simulink model "BD_SER2"  (Simulink 4.1.1)
settings: Solver=ode1  SolverMode=SingleTasking  StartTime=0.0  StopTime=max(cyc_mph(:,1))  FixedStep=1  MaxStep=1  RelTol=1e-3  AbsTol=1e-3
undefined symbols (not defined in the file): air_cp, amb_tmp, cyc_avg_time, cyc_cargo_mass, cyc_elevation_init, cyc_filter_bool, cyc_grade, cyc_mph, enable_stop, ess_cap_scale, ess_coulombic_eff, ess_init_soc, ess_max_ah_cap, ess_max_volts, ess_min_volts, ess_mod_airflow, ess_mod_cp, ess_mod_init_tmp, ess_module_mass, ess_module_num, ess_on, ess_res_scale_coef, ess_res_scale_fun, ess_set_tmp, ess_th_calc, ess_th_res_off, ess_th_res_on, ess_tmp, ess_voc, ex_calc, fc_ct_trq, fc_emis, fc_inertia, fc_map_spd, fc_max_trq, fc_spd_scale, fc_trq_scale, fd_inertia, fd_loss, fd_ratio, gb_dnshift_load, gb_dnshift_spd, gb_gears_num, gb_inertia, gb_num_init, gb_ratio, gb_shift_delay, gb_spd_scale, gb_trq_scale, gb_upshift_load, gb_upshift_spd, gc_inertia, gc_map_spd, gc_map_trq, gc_max_crrnt, gc_max_trq, gc_outpwr_map, gc_overtrq_factor, gc_spd_scale, gc_trq_scale ... (+37)
libraries: lib_wheel2 x12, lib_accessory2 x4, lib_controls2 x3, lib_etc x2, lib_help x2, lib_fuel_converter x2, lib_drive_cycle2 x1, lib_interactive x1, lib_drive_cycle x1, lib_exhaust x1, lib_fuel_converter3 x1
(part 11 of 15)

== system BD_SER2/final drive <fd>/model&interface/model/enhancedToWorkspace4 ==
  In1 : Inport  Port=1  LatchInput=off
  To Workspace : ToWorkspace  VariableName=fd_spd_in_r  SampleTime=-1  SaveFormat=Array
  wires:
  In1/1 -> To Workspace/1

== system BD_SER2/final drive <fd>/model&interface/model/enhancedToWorkspace5 ==
  In1 : Inport  Port=1  LatchInput=off
  To Workspace : ToWorkspace  VariableName=fd_trq_in_r  SampleTime=-1  SaveFormat=Array
  wires:
  In1/1 -> To Workspace/1

== system BD_SER2/final drive <fd>/model&interface/model/enhancedToWorkspace6 ==
  In1 : Inport  Port=1  LatchInput=off
  To Workspace : ToWorkspace  VariableName=fd_trq_out_r  SampleTime=-1  SaveFormat=Array
  wires:
  In1/1 -> To Workspace/1

== system BD_SER2/final drive <fd>/model&interface/model/enhancedToWorkspace7 ==
  In1 : Inport  Port=1  LatchInput=off
  To Workspace : ToWorkspace  VariableName=fd_spd_out_r  SampleTime=-1  SaveFormat=Array
  wires:
  In1/1 -> To Workspace/1

== system BD_SER2/final drive <fd>/model&interface/model/help ==

== system BD_SER2/final drive <fd>/model&interface/model/loss (Nm) ==
  note: The loss torque is zero when the gears are not turning,
      | and is applied at the input side of the gear reduction.
  fd output speed (rad/s) : Inport  Port=1  LatchInput=off
  Constant : Constant  Orientation=up  Value=0
  Switch : Switch  Threshold=eps
  final drive loss torque (Nm) : Constant  Value=fd_loss
  drag torque (Nm) : Outport  Port=1  InitialOutput=0
  wires:
  Constant/1 -> Switch/3
  fd output speed (rad/s)/1 -> Switch/2
  Switch/1 -> drag torque (Nm)/1
  final drive loss torque (Nm)/1 -> Switch/1

== system BD_SER2/fuel converter  <fc> for series/Model & Interface/model/Block NOTES ==
  note: This block models the internal combustion engine, and includes inertia effects,
      | performance limits, accessory loads, and temperature transient effects on fuel
      | use, engine-out emissions, and catalyst efficiency.  There are 'leads' to the
      | engine controller here, which controller determines whether the engine is on.

== system BD_SER2/fuel converter  <fc> for series/Model & Interface/model/enhancedToWorkspace ==
  In1 : Inport  Port=1  LatchInput=off
  To Workspace : ToWorkspace  VariableName=fc_spd_out_r  SampleTime=-1  SaveFormat=Array
  wires:
  In1/1 -> To Workspace/1

== system BD_SER2/fuel converter  <fc> for series/Model & Interface/model/enhancedToWorkspace1 ==
  In1 : Inport  Port=1  LatchInput=off
  To Workspace : ToWorkspace  VariableName=fc_trq_out_r  SampleTime=-1  SaveFormat=Array
  wires:
  In1/1 -> To Workspace/1

== system BD_SER2/fuel converter  <fc> for series/Model & Interface/model/enhancedToWorkspace2 ==
  In1 : Inport  Port=1  LatchInput=off
  To Workspace : ToWorkspace  VariableName=fc_spd_est  SampleTime=-1  SaveFormat=Array
  wires:
  In1/1 -> To Workspace/1

== system BD_SER2/fuel converter  <fc> for series/Model & Interface/model/enhancedToWorkspace3 ==
  In1 : Inport  Port=1  LatchInput=off
  To Workspace : ToWorkspace  VariableName=fc_brake_trq  SampleTime=-1  SaveFormat=Array
  wires:
  In1/1 -> To Workspace/1

== system BD_SER2/fuel converter  <fc> for series/Model & Interface/model/enhancedToWorkspace4 ==
  In1 : Inport  Port=1  LatchInput=off
  To Workspace : ToWorkspace  VariableName=fc_trq_out_a  SampleTime=-1  SaveFormat=Array
  wires:
  In1/1 -> To Workspace/1

== system BD_SER2/fuel converter  <fc> for series/Model & Interface/model/enhancedToWorkspace5 ==
  In1 : Inport  Port=1  LatchInput=off
  To Workspace : ToWorkspace  VariableName=fc_spd_out_a  SampleTime=-1  SaveFormat=Array
  wires:
  In1/1 -> To Workspace/1

== system BD_SER2/fuel converter  <fc> for series/Model & Interface/model/fuel use and EO emis Configurable Subsystem ==
  T (Nm) : Inport  Port=1  LatchInput=off
  w (rad/s) : Inport  Port=2  LatchInput=off
  fuel use and EO emis : lib_fuel_converter3/configurable subsystems/fuel use and EO emis
      settings: RTWFcnNameOpts=Auto  RTWFileNameOpts=Auto
  cumulative fuel  use (gal) : Outport  Port=1
  "FC ON?, EOem, MFex, Tex, O2ex" : Outport  Port=2
  Vv,Tfc : Outport  Port=3
  wires:
  T (Nm)/1 -> fuel use and EO emis/1
  w (rad/s)/1 -> fuel use and EO emis/2
  fuel use and EO emis/1 -> cumulative fuel  use (gal)/1
  fuel use and EO emis/2 -> "FC ON?, EOem, MFex, Tex, O2ex"/1
  fuel use and EO emis/3 -> Vv,Tfc/1

== system BD_SER2/fuel converter  <fc> for series/Model & Interface/model/help ==

== system BD_SER2/fuel converter  <fc> for series/Model & Interface/model/providing trq (+ive or -ive) ==
  req'd trq (Nm) : Inport  Port=1  LatchInput=off
  req'd spd (rad/s) : Inport  Port=2  LatchInput=off
  prev engine spd (rad/s) : Inport  Port=3  LatchInput=off
  Mux3 : Mux  Inputs=3
      settings: DisplayOption=none
  Sum1 : Sum  Inputs=+-  SaturateOnIntegerOverflow=on
  Sum2 : Sum  Inputs=++  SaturateOnIntegerOverflow=on
  effect of inertia (Nm) : Subsystem
      settings: RTWFcnNameOpts=Auto  RTWFileNameOpts=Auto
  enforce engine limits : Subsystem
      settings: RTWFcnNameOpts=Auto  RTWFileNameOpts=Auto
  map trq (Nm) spd (rad/s) trq to drivetrain (Nm) : Outport  Port=1  InitialOutput=0
  wires:
  Sum2/1 -> enforce engine limits/1(req'd engine trq (Nm))
  effect of inertia (Nm)/1((Nm)) -> Sum2/2, Sum1/2
  req'd trq (Nm)/1 -> Sum2/1
  enforce engine limits/2(limited engine spd (rad/s)) -> Mux3/2, effect of inertia (Nm)/1(req'd spd (rad/s))
  enforce engine limits/1(limited engine brake trq (Nm)) -> Sum1/1, Mux3/1
  prev engine spd (rad/s)/1 -> effect of inertia (Nm)/2(prev spd)
  Mux3/1 -> map trq (Nm) spd (rad/s) trq to drivetrain (Nm)/1
  Sum1/1 -> Mux3/3
  req'd spd (rad/s)/1 -> enforce engine limits/2(req'd engine spd (rad/s))

== system BD_SER2/fuel converter  <fc> for series/Model & Interface/model/spinning up or spinning down ==
  spd command (rad/s) : Inport  Port=1  LatchInput=off
  engine disconnected from drivetrain : Inport  Port=2  LatchInput=off
  previous engine spd (rad/s) : Inport  Port=3  LatchInput=off
  Constant : Constant  Value=0
  Constant1 : Constant  Value=vc_idle_spd
  MinMax : MinMax  Function=min  Inputs=2
  MinMax1 : MinMax  Function=max  Inputs=2
  Mux3 : Mux  Inputs=3
      settings: DisplayOption=none
  Product : Product  Inputs=2  Multiplication=Element-wise(.*)  SaturateOnIntegerOverflow=on
  Product2 : Product  Inputs=2  Multiplication=Element-wise(.*)  SaturateOnIntegerOverflow=on
  Relational Operator : RelationalOperator  Operator=<=
  Sum : Sum  Inputs=|++  SaturateOnIntegerOverflow=on
  Sum1 : Sum  Inputs=|+-  SaturateOnIntegerOverflow=on
  Sum2 : Sum  Inputs=++  SaturateOnIntegerOverflow=on
  Switch: map torque : Switch  Threshold=eps
  T_closed throttle : Subsystem
      settings: RTWFcnNameOpts=Auto  RTWFileNameOpts=Auto
  T_max : Subsystem
      settings: RTWFcnNameOpts=Auto  RTWFileNameOpts=Auto
  alpha : Gain  Gain=1/(fc_inertia+eps)  Multiplication=Element-wise(K.*u)  SaturateOnIntegerOverflow=on
  dt : Subsystem
      settings: RTWFcnNameOpts=Auto  RTWFileNameOpts=Auto
  effect of inertia (Nm) : Subsystem
      settings: RTWFcnNameOpts=Auto  RTWFileNameOpts=Auto
  just started spin-down/spin-up : Subsystem
      settings: RTWFcnNameOpts=Auto  RTWFileNameOpts=Auto
  no-lag Reset Integrator : Subsystem  mask(No-lag Reset Integrator){@1=vc_idle_spd}
      mask prompts: @1 "Initial Value"
      mask help: No-lag Reset Integrator
      mask init:
      | initval=@1;
      settings: RTWFcnNameOpts=Auto  RTWFileNameOpts=Auto
      mask Help: Integrates first input using Euler technique.\nAt the time step that input 2 <> zero,\noutput is reset to input 3.
      mask Display: disp('1/s\nw/ reset\nno lag')
  map trq (Nm) spd (rad/s) trq to drivetrain (Nm) : Outport  Port=1  InitialOutput=0
  wires:
  T_max/1(T_max) -> MinMax/1
  MinMax/1 -> Switch: map torque/1
  T_closed throttle/1(T_closed throttle) -> Switch: map torque/3
  Switch: map torque/1 -> Mux3/1, Sum1/1
  Relational Operator/1 -> Switch: map torque/2
  alpha/1 -> Product/1, no-lag Reset Integrator/1(in_1)
  previous engine spd (rad/s)/1 -> T_closed throttle/1(w_APU), T_max/1(w_APU), effect of inertia (Nm)/2(prev spd), Relational Operator/1, Sum2/2
  spd command (rad/s)/1 -> Relational Operator/2, effect of inertia (Nm)/1(req'd spd (rad/s))
  no-lag Reset Integrator/1(out_1) -> MinMax1/1
  just started spin-down/spin-up/1(trigger) -> no-lag Reset Integrator/2(in_2)
  Sum2/1 -> no-lag Reset Integrator/3(in_3)
  engine disconnected from drivetrain/1 -> just started spin-down/spin-up/1(state)
  Product/1 -> Sum2/1
  dt/1(out_1) -> Product/2
  Mux3/1 -> map trq (Nm) spd (rad/s) trq to drivetrain (Nm)/1
  Constant/1 -> Mux3/3
  Constant1/1 -> Product2/1
  [engine_on] -> Product2/2
  Product2/1 -> MinMax1/2
  MinMax1/1 -> Mux3/2
  effect of inertia (Nm)/1((Nm)) -> Sum/1
  Sum/1 -> MinMax/2
  [acc_mech_trq_est] -> Sum/2
  Sum1/1 -> alpha/1
  [acc_mech_trq_est] -> Sum1/2

== system BD_SER2/gearbox <gb> old/gearbox model & interface/gearbox model/Block NOTES ==
  note: This is a good assumption, at least for the VW 4-speed manual transaxle of SAE 820741.
      | In the VW transaxle, efficiency is fairly independent of torque and speed at high torques.
  note: Available output torque is estimated assuming that the gearbox efficiency for theavailable input
      | torque andspeed is the same as the gearbox efficiency for the REQUESTED input torque.
  note: The inertia torque is the input torque required to accelerate the
      | final drive's inertia as measured on the input side.
  note: The loss torque is zero when the gears are not turning,
      | and is applied at the input side of the gear reduction.
  note: This gearbox model includes loss data, rotational inertia, and a gear reduction.

== system BD_SER2/gearbox <gb> old/gearbox model & interface/gearbox model/Pout/Pin neglecting inertia ==
  note: Pout/Pin, neglecting inertia, is used to estimate the output torque given the
      | input torque in a very simple forward-facing calculation.
  Tin : Inport  Port=1  LatchInput=off
  Tinertia : Inport  Port=2  LatchInput=off
  Tout : Inport  Port=3  LatchInput=off
  gear ratio : Inport  Port=4  LatchInput=off
  Constant1 : Constant  Orientation=up  Value=0
  Pout/Pin (neglecting inertia) : Subsystem
      settings: RTWFcnNameOpts=Auto  RTWFileNameOpts=Auto
      mask Display: disp('/')
  Product : Product  Inputs=2  Multiplication=Element-wise(.*)  SaturateOnIntegerOverflow=on
  Relational Operator : RelationalOperator  Operator=~=
  Saturation : Saturate  UpperLimit=inf  LowerLimit=0  LinearizeAsGain=on
  Switch : Switch  Threshold=eps
  Tin-Tinertia : Sum  Inputs=+-  SaturateOnIntegerOverflow=on
  make division bombproof : Subsystem
      settings: RTWFcnNameOpts=Auto  RTWFileNameOpts=Auto
  Pout/Pin : Outport  Port=1  InitialOutput=0
  wires:
  gear ratio/1 -> Product/1
  Product/1 -> Pout/Pin (neglecting inertia)/2(in_2)
  Tout/1 -> Pout/Pin (neglecting inertia)/1(in_1)
  Tin-Tinertia/1 -> make division bombproof/1(Tin-Tinertia), Relational Operator/1
  Saturation/1 -> Pout/Pin/1
  Switch/1 -> Saturation/1
  Relational Operator/1 -> Switch/2
  Pout/Pin (neglecting inertia)/1(out_1) -> Switch/1
  Tin/1 -> Tin-Tinertia/1
  Tinertia/1 -> Tin-Tinertia/2
  make division bombproof/1(Out1) -> Product/2
  Constant1/1 -> Relational Operator/2, Switch/3

== system BD_SER2/gearbox <gb> old/gearbox model & interface/gearbox model/effect of inertia (Nm) ==
  note: The inertia torque is the input torque required to accelerate the
      | gearbox's inertia as measured on the input side.
  gb input speed (rad/s) : Inport  Port=1  LatchInput=off
  Gain : Gain  Gain=gb_inertia  Multiplication=Element-wise(K.*u)  SaturateOnIntegerOverflow=on
  d/dt : Derivative
  drag torque (Nm) : Outport  Port=1  InitialOutput=0
  wires:
  gb input speed (rad/s)/1 -> d/dt/1
  d/dt/1 -> Gain/1
  Gain/1 -> drag torque (Nm)/1

== system BD_SER2/gearbox <gb> old/gearbox model & interface/gearbox model/enhancedToWorkspace ==
  In1 : Inport  Port=1  LatchInput=off
  To Workspace : ToWorkspace  VariableName=gb_spd_in_a  SampleTime=-1  SaveFormat=Array
  wires:
  In1/1 -> To Workspace/1

== system BD_SER2/gearbox <gb> old/gearbox model & interface/gearbox model/enhancedToWorkspace1 ==
  In1 : Inport  Port=1  LatchInput=off
  To Workspace : ToWorkspace  VariableName=gb_trq_in_a  SampleTime=-1  SaveFormat=Array
  wires:
  In1/1 -> To Workspace/1

== system BD_SER2/gearbox <gb> old/gearbox model & interface/gearbox model/enhancedToWorkspace2 ==
  In1 : Inport  Port=1  LatchInput=off
  To Workspace : ToWorkspace  VariableName=gb_spd_out_a  SampleTime=-1  SaveFormat=Array
  wires:
  In1/1 -> To Workspace/1

== system BD_SER2/gearbox <gb> old/gearbox model & interface/gearbox model/enhancedToWorkspace3 ==
  In1 : Inport  Port=1  LatchInput=off
  To Workspace : ToWorkspace  VariableName=gb_trq_out_a  SampleTime=-1  SaveFormat=Array
  wires:
  In1/1 -> To Workspace/1

== system BD_SER2/gearbox <gb> old/gearbox model & interface/gearbox model/enhancedToWorkspace4 ==
  In1 : Inport  Port=1  LatchInput=off
  To Workspace : ToWorkspace  VariableName=gb_ni_trq_out_a  SampleTime=-1  SaveFormat=Array
  wires:
  In1/1 -> To Workspace/1

== system BD_SER2/gearbox <gb> old/gearbox model & interface/gearbox model/enhancedToWorkspace5 ==
  In1 : Inport  Port=1  LatchInput=off
  To Workspace : ToWorkspace  VariableName=gb_spd_in_r  SampleTime=-1  SaveFormat=Array
  wires:
  In1/1 -> To Workspace/1

== system BD_SER2/gearbox <gb> old/gearbox model & interface/gearbox model/enhancedToWorkspace6 ==
  In1 : Inport  Port=1  LatchInput=off
  To Workspace : ToWorkspace  VariableName=gb_trq_in_r  SampleTime=-1  SaveFormat=Array
  wires:
  In1/1 -> To Workspace/1

== system BD_SER2/gearbox <gb> old/gearbox model & interface/gearbox model/enhancedToWorkspace7 ==
  In1 : Inport  Port=1  LatchInput=off
  To Workspace : ToWorkspace  VariableName=gb_spd_out_r  SampleTime=-1  SaveFormat=Array
  wires:
  In1/1 -> To Workspace/1

== system BD_SER2/gearbox <gb> old/gearbox model & interface/gearbox model/enhancedToWorkspace8 ==
  In1 : Inport  Port=1  LatchInput=off
  To Workspace : ToWorkspace  VariableName=gb_trq_out_r  SampleTime=-1  SaveFormat=Array
  wires:
  In1/1 -> To Workspace/1

== system BD_SER2/gearbox <gb> old/gearbox model & interface/gearbox model/enhancedToWorkspace9 ==
  In1 : Inport  Port=1  LatchInput=off
  To Workspace : ToWorkspace  VariableName=gb_gear_number  SampleTime=-1  SaveFormat=Array
  wires:
  In1/1 -> To Workspace/1

== system BD_SER2/gearbox <gb> old/gearbox model & interface/gearbox model/gearbox controller interface ==
  T_gb_out : Inport  Port=1  LatchInput=off
  w_gb_out : Inport  Port=2  LatchInput=off
  eta_gb : Inport  Port=3  LatchInput=off
  enhancedToWorkspace1 : Subsystem  mask(enhancedToWorkspace){generalName=generalName, specificName=gear_ratio, logFlag=logFlag}
      mask prompts: generalName "General Name [char-evaluated]"; specificName "Specific Name [char-literal]"; logFlag "Enable flag (1=on,0=off)"
      mask help: A wrapper for the Simulink "To Workspace" block that allows you to evaluate the name of the variable to log to workspace. This is useful to avoid the double logging errors that occur when you pull in two library models that attempt to log to the same variable.
      mask init:
      | enhancedToWsMaker
      settings: CopyFcn=breakLinkCopyFcn  ParentCloseFcn=breakLinkParCloseFcn  RTWFcnNameOpts=Auto  RTWFileNameOpts=Auto
      mask Help:
      | <h2>Enhanced To Workspace Block</h2>
      | <h3>Parameters</h3>
      | <UL>
      | <li><b>General Name:</b> This is the more general name of the variable. Variables are saved to the workspace as <i>generalName_specificName</i>. Note that this is an evaluated variable. If you would like to type in the value directly, it must be surrounded with single quotes. Otherwise you can input the name of a variable containing a char string.</li>
      | <li><b>Specific Name:</b> This is the specific name of the variable. Note that this is input as a char literal (i.e., you don't need quotes).</li>
      | <li><b>Enable Flag:</b> This flag should have the value of 0 or 1. If 0, the variable will not be logged to the workspace. If 1, the variable will be logged. This is done so that variable logging can be turned off to improve speed.</li>
      | </ul>
      | <h3>Overview</h3>
      | <p>The enhanced to workspace block was put together to allow one to dynamically resolve variable names at run time in simulink. This is most powerful when used in conjunction with a masked subsystem to allow multiple instances of that masked subsytem to be used in the same model. The strategy is to set the generalName in the block mask which will allow the block to change the general name for all variable logging on the fly.
      | <h3>Helper Files</h3>
      | <p>Three m-files are required by the enhancedToWorkspace block. These files are located in the &lt; ADVISOR root &gt;/GUI directory :
      | <ul>
      | <li><i>enhancedToWsMaker.m</i> This file runs the mask initialization for the block</li>
      | <li><i>breakLinkCopyFcn.m</i> This file is used by the block callback when the simulink block is copied. It is necessary to break the link to the enhancedToWorkspace similar to the To Workspace block in order for it to be able to configure itself. (Try copying simulink's To Workspace block--it is impossible to make a link)</li>
      | <li><i>breakLinkParCloseFcn.m</i> This file is similar to the breakLinkCopyFcn and is used when a parent system is closed</li>
      | </ul>
      | <hr>
      | 
      | <p>Created 2003-Jan-21, Michael Patrick O'Keefe, NREL</p>
      mask Display: disp([generalName,'_',specificName])
  enhancedToWorkspace8 : Subsystem  mask(enhancedToWorkspace){generalName=generalName, specificName=shifting, logFlag=logFlag}
      mask prompts: generalName "General Name [char-evaluated]"; specificName "Specific Name [char-literal]"; logFlag "Enable flag (1=on,0=off)"
      mask help: A wrapper for the Simulink "To Workspace" block that allows you to evaluate the name of the variable to log to workspace. This is useful to avoid the double logging errors that occur when you pull in two library models that attempt to log to the same variable.
      mask init:
      | enhancedToWsMaker
      settings: CopyFcn=breakLinkCopyFcn  ParentCloseFcn=breakLinkParCloseFcn  RTWFcnNameOpts=Auto  RTWFileNameOpts=Auto
      mask Help:
      | <h2>Enhanced To Workspace Block</h2>
      | <h3>Parameters</h3>
      | <UL>
      | <li><b>General Name:</b> This is the more general name of the variable. Variables are saved to the workspace as <i>generalName_specificName</i>. Note that this is an evaluated variable. If you would like to type in the value directly, it must be surrounded with single quotes. Otherwise you can input the name of a variable containing a char string.</li>
      | <li><b>Specific Name:</b> This is the specific name of the variable. Note that this is input as a char literal (i.e., you don't need quotes).</li>
      | <li><b>Enable Flag:</b> This flag should have the value of 0 or 1. If 0, the variable will not be logged to the workspace. If 1, the variable will be logged. This is done so that variable logging can be turned off to improve speed.</li>
      | </ul>
      | <h3>Overview</h3>
      | <p>The enhanced to workspace block was put together to allow one to dynamically resolve variable names at run time in simulink. This is most powerful when used in conjunction with a masked subsystem to allow multiple instances of that masked subsytem to be used in the same model. The strategy is to set the generalName in the block mask which will allow the block to change the general name for all variable logging on the fly.
      | <h3>Helper Files</h3>
      | <p>Three m-files are required by the enhancedToWorkspace block. These files are located in the &lt; ADVISOR root &gt;/GUI directory :
      | <ul>
      | <li><i>enhancedToWsMaker.m</i> This file runs the mask initialization for the block</li>
      | <li><i>breakLinkCopyFcn.m</i> This file is used by the block callback when the simulink block is copied. It is necessary to break the link to the enhancedToWorkspace similar to the To Workspace block in order for it to be able to configure itself. (Try copying simulink's To Workspace block--it is impossible to make a link)</li>
      | <li><i>breakLinkParCloseFcn.m</i> This file is similar to the breakLinkCopyFcn and is used when a parent system is closed</li>
      | </ul>
      | <hr>
      | 
      | <p>Created 2003-Jan-21, Michael Patrick O'Keefe, NREL</p>
      mask Display: disp([generalName,'_',specificName])
  gear_ratio : Outport  Port=1  InitialOutput=0
  shifting : Outport  Port=2  InitialOutput=0
  tag scope: T_gb_out=scoped, eta_gb=scoped, w_gb_out=scoped
  wires:
  [shifting] -> enhancedToWorkspace8/1(In1), shifting/1
  T_gb_out/1 -> [T_gb_out]
  w_gb_out/1 -> [w_gb_out]
  eta_gb/1 -> [eta_gb]
  [gear_ratio] -> enhancedToWorkspace1/1(In1), gear_ratio/1

== system BD_SER2/gearbox <gb> old/gearbox model & interface/gearbox model/gearing (Nm) (rad/s) ==
  "output shaft torque and speed  (Nm), (rad/s)" : Inport  Port=1  LatchInput=off
  gear ratio : Inport  Port=2  LatchInput=off
  Demux : Demux  Outputs=2  BusSelectionMode=off
  Fcn1 : Fcn  Expr=1/u
  Product2 : Product  Inputs=2  Multiplication=Element-wise(.*)  SaturateOnIntegerOverflow=on
  Product3 : Product  Inputs=2  Multiplication=Element-wise(.*)  SaturateOnIntegerOverflow=on
  input shaft torque (Nm) : Outport  Port=1  InitialOutput=0
  input shaft speed (rad/s) : Outport  Port=2  InitialOutput=0
  wires:
  Demux/2 -> Product3/1
  Demux/1 -> Product2/1
  gear ratio/1 -> Product3/2, Fcn1/1
  "output shaft torque and speed  (Nm), (rad/s)"/1 -> Demux/1
  Fcn1/1 -> Product2/2
  Product2/1 -> input shaft torque (Nm)/1
  Product3/1 -> input shaft speed (rad/s)/1

== system BD_SER2/gearbox <gb> old/gearbox model & interface/gearbox model/gearing (Nm) (rad/s)1 ==
  input shaft torque (Nm) : Inport  Port=1  LatchInput=off
  input shaft speed (rad/s) : Inport  Port=2  LatchInput=off
  gear ratio : Inport  Port=3  LatchInput=off
  Fcn1 : Fcn  Expr=1/u
  Product2 : Product  Inputs=2  Multiplication=Element-wise(.*)  SaturateOnIntegerOverflow=on
  Product3 : Product  Inputs=2  Multiplication=Element-wise(.*)  SaturateOnIntegerOverflow=on
  output shaft torque (Nm) : Outport  Port=1  InitialOutput=0
  output shaft speed (rad/s) : Outport  Port=2  InitialOutput=0
  wires:
  input shaft speed (rad/s)/1 -> Product3/2
  input shaft torque (Nm)/1 -> Product2/1
  Product2/1 -> output shaft torque (Nm)/1
  Product3/1 -> output shaft speed (rad/s)/1
  gear ratio/1 -> Fcn1/1, Product2/2
  Fcn1/1 -> Product3/1

== system BD_SER2/gearbox <gb> old/gearbox model & interface/gearbox model/help ==

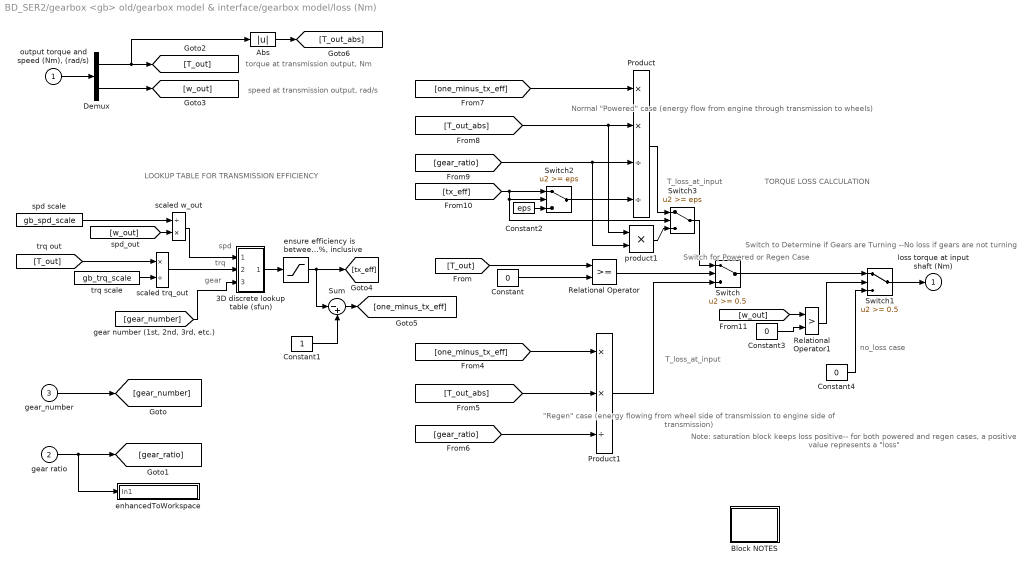
== system BD_SER2/gearbox <gb> old/gearbox model & interface/gearbox model/loss (Nm) ==
  note: LOOKUP TABLE FOR TRANSMISSION EFFICIENCY
  note: T_loss_at_input
  note: "Regen" case
      | (energy flowing from
      | wheel side of transmission
      | to engine side of transmission)
  note: T_loss_at_input
  note: Normal "Powered" case
      | (energy flow from engine
      | through transmission to wheels)
  note: Switch to Determine
      | if Gears are Turning
      | --No loss if gears
      | are not turning
  note: Switch for Powered
      |  or Regen Case
  note: Note: saturation block keeps
      | loss positive-- for both powered
      | and regen cases, a
      | positive value represents a "loss"
  note: no_loss case
  note: speed at transmission output, rad/s
  note: torque at transmission output, Nm
  note: spd
  note: trq
  note: gear
  note: TORQUE LOSS CALCULATION
  "output torque and speed (Nm), (rad/s)" : Inport  Port=1  LatchInput=off
  gear ratio : Inport  Port=2  LatchInput=off
  gear_number : Inport  Port=3  LatchInput=off
  3D discrete lookup table (sfun) : Subsystem  mask{tx_map_spd=tx_map_spd, tx_map_trq=tx_map_trq, tx_eff_map=tx_eff_map}
      mask prompts: tx_map_spd "Row Lookup"; tx_map_trq "Column Lookup"; tx_eff_map "Lookup Matrix"
      settings: RTWFcnNameOpts=Auto  RTWFileNameOpts=Auto
  Abs : Abs  SaturateOnIntegerOverflow=on
  Block NOTES : Subsystem
      settings: RTWFcnNameOpts=Auto  RTWFileNameOpts=Auto
      mask Display: disp('Block\nNOTES')
  Constant : Constant  Value=0
  Constant1 : Constant  Value=1
  Constant2 : Constant  Value=eps
  Constant3 : Constant  Value=0
  Constant4 : Constant  Value=0
  Demux : Demux  Outputs=2  BusSelectionMode=off
  Product : Product  Inputs=**//  Multiplication=Element-wise(.*)  SaturateOnIntegerOverflow=on
  Product1 : Product  Inputs=**/  Multiplication=Element-wise(.*)  SaturateOnIntegerOverflow=on
  Relational Operator : RelationalOperator  Operator=>=
  Relational Operator1 : RelationalOperator  Operator=>
  Sum : Sum  Inputs=|-+  SaturateOnIntegerOverflow=on
  Switch : Switch  Threshold=0.5
  Switch1 : Switch  Threshold=0.5
  Switch2 : Switch  Threshold=eps
  Switch3 : Switch  Threshold=eps
  enhancedToWorkspace : Subsystem  TreatAsAtomicUnit=on  mask(enhancedToWorkspace){generalName=generalName, specificName=current_gear_ratio, logFlag=logFlag}
      mask prompts: generalName "General Name [char-evaluated]"; specificName "Specific Name [char-literal]"; logFlag "Enable flag (1=on,0=off)"
      mask help: A wrapper for the Simulink "To Workspace" block that allows you to evaluate the name of the variable to log to workspace. This is useful to avoid the double logging errors that occur when you pull in two library models that attempt to log to the same variable.
      mask init:
      | enhancedToWsMaker
      settings: CopyFcn=breakLinkCopyFcn  ParentCloseFcn=breakLinkParCloseFcn  RTWFcnNameOpts=Auto  RTWFileNameOpts=Auto
      mask Help:
      | <h2>Enhanced To Workspace Block</h2>
      | <h3>Parameters</h3>
      | <UL>
      | <li><b>General Name:</b> This is the more general name of the variable. Variables are saved to the workspace as <i>generalName_specificName</i>. Note that this is an evaluated variable. If you would like to type in the value directly, it must be surrounded with single quotes. Otherwise you can input the name of a variable containing a char string.</li>
      | <li><b>Specific Name:</b> This is the specific name of the variable. Note that this is input as a char literal (i.e., you don't need quotes).</li>
      | <li><b>Enable Flag:</b> This flag should have the value of 0 or 1. If 0, the variable will not be logged to the workspace. If 1, the variable will be logged. This is done so that variable logging can be turned off to improve speed.</li>
      | </ul>
      | <h3>Overview</h3>
      | <p>The enhanced to workspace block was put together to allow one to dynamically resolve variable names at run time in simulink. This is most powerful when used in conjunction with a masked subsystem to allow multiple instances of that masked subsytem to be used in the same model. The strategy is to set the generalName in the block mask which will allow the block to change the general name for all variable logging on the fly.
      | <h3>Helper Files</h3>
      | <p>Three m-files are required by the enhancedToWorkspace block. These files are located in the &lt; ADVISOR root &gt;/GUI directory :
      | <ul>
      | <li><i>enhancedToWsMaker.m</i> This file runs the mask initialization for the block</li>
      | <li><i>breakLinkCopyFcn.m</i> This file is used by the block callback when the simulink block is copied. It is necessary to break the link to the enhancedToWorkspace similar to the To Workspace block in order for it to be able to configure itself. (Try copying simulink's To Workspace block--it is impossible to make a link)</li>
      | <li><i>breakLinkParCloseFcn.m</i> This file is similar to the breakLinkCopyFcn and is used when a parent system is closed</li>
      | </ul>
      | <hr>
      | 
      | <p>Created 2003-Jan-21, Michael Patrick O'Keefe, NREL</p>
      | 
      | <!--
      | <VARDEF>
      | <H3>var_name</H3>
      | <UL>
      | <LI><B>data type</B> data type here</LI>
      | <LI><B>units</B> units here</LI>
      | <LI><B>vehicle type</B> vehicle type here</LI>
      | <LI><B>description</B> description here</LI>
      | </UL>
      | </VARDEF>
      | -->
      mask Display: disp([generalName,'_',specificName])
  "ensure efficiency is between  0% and 100%, inclusive" : Saturate  UpperLimit=1  LowerLimit=0  LinearizeAsGain=on
  product1 : Product  Inputs=2  Multiplication=Element-wise(.*)  SaturateOnIntegerOverflow=on
  scaled trq_out : Product  Inputs=*/  Multiplication=Element-wise(.*)  SaturateOnIntegerOverflow=on
  scaled w_out : Product  Inputs=/*  Multiplication=Element-wise(.*)  SaturateOnIntegerOverflow=on
  spd scale : Constant  Value=gb_spd_scale
  trq scale : Constant  Value=gb_trq_scale
  loss torque at input shaft (Nm) : Outport  Port=1  InitialOutput=0
  wires:
  "output torque and speed (Nm), (rad/s)"/1 -> Demux/1
  Demux/2 -> [w_out]
  [gear_number] -> 3D discrete lookup table (sfun)/3("gear_number  (e.g., 1, 2, 3)")
  Relational Operator/1 -> Switch/2
  Constant/1 -> Relational Operator/2
  [T_out] -> Relational Operator/1
  Product1/1 -> Switch/3
  [one_minus_tx_eff] -> Product1/1
  [gear_ratio] -> Product1/3
  [T_out_abs] -> Product1/2
  [one_minus_tx_eff] -> Product/1
  [T_out_abs] -> Product/2, product1/1
  [gear_ratio] -> Product/3, product1/2
  Switch1/1 -> loss torque at input shaft (Nm)/1
  Constant4/1 -> Switch1/3
  [w_out] -> Relational Operator1/1
  Constant3/1 -> Relational Operator1/2
  Relational Operator1/1 -> Switch1/2
  Demux/1 -> [T_out], Abs/1
  Abs/1 -> [T_out_abs]
  Switch/1 -> Switch1/1
  3D discrete lookup table (sfun)/1(tx_eff) -> "ensure efficiency is between  0% and 100%, inclusive"/1
  "ensure efficiency is between  0% and 100%, inclusive"/1 -> [tx_eff], Sum/1
  scaled w_out/1 -> 3D discrete lookup table (sfun)/1(lookup speed (rad/s))
  [T_out] -> scaled trq_out/1
  scaled trq_out/1 -> 3D discrete lookup table (sfun)/2(lookup trq (Nm))
  trq scale/1 -> scaled trq_out/2
  Constant1/1 -> Sum/2
  Sum/1 -> [one_minus_tx_eff]
  [w_out] -> scaled w_out/2
  spd scale/1 -> scaled w_out/1
  gear ratio/1 -> enhancedToWorkspace/1(In1), [gear_ratio]
  gear_number/1 -> [gear_number]
  Switch2/1 -> Product/4
  [tx_eff] -> Switch2/1, Switch2/2, Switch3/2
  Constant2/1 -> Switch2/3
  Switch3/1 -> Switch/1
  Product/1 -> Switch3/1
  product1/1 -> Switch3/3

== system BD_SER2/generator/ controller <gc>/GC Model/model/Block NOTES ==
  note: This generator/controller model includes loss data, rotational inertia, and performance limits.
      | This is the only entirely forward-facing block in ADVISOR, computing the output power from the
      | input torque and speed.  The generator map used in the lookup table block is VERY similar to
      | the input power motor map, with the main difference being that the torque and power sign
      | conventions are opposite: here torque input to the machine and power output by the machine
      | are positive.

== system BD_SER2/generator/ controller <gc>/GC Model/model/effect of inertia (Nm) ==
  in_1 : Inport  Port=1  LatchInput=off
  Gain : Gain  Gain=gc_inertia  Multiplication=Element-wise(K.*u)  SaturateOnIntegerOverflow=on
  alpha : Derivative
  out_1 : Outport  Port=1  InitialOutput=0
  wires:
  in_1/1 -> alpha/1
  alpha/1 -> Gain/1
  Gain/1 -> out_1/1

== system BD_SER2/generator/ controller <gc>/GC Model/model/enforce torque limit ==
  req'd generator input torque (Nm) : Inport  Port=1  LatchInput=off
  limited generator speed (rad/s) : Inport  Port=2  LatchInput=off
  Block NOTES : Subsystem
      settings: RTWFcnNameOpts=Auto  RTWFileNameOpts=Auto
      mask Display: disp('Block\nNOTES')
  MinMax : MinMax  Function=min  Inputs=2
  max torque : Lookup  InputValues=gc_map_spd*gc_spd_scale  OutputValues=gc_max_trq*gc_overtrq_factor*gc_trq_scale
  limited generator input torque (Nm) : Outport  Port=1
  wires:
  req'd generator input torque (Nm)/1 -> MinMax/1
  max torque/1 -> MinMax/2
  MinMax/1 -> limited generator input torque (Nm)/1
  limited generator speed (rad/s)/1 -> max torque/1

== system BD_SER2/generator/ controller <gc>/GC Model/model/enhancedToWorkspace ==
  In1 : Inport  Port=1  LatchInput=off
  To Workspace : ToWorkspace  VariableName=gc_pwr_out_a  SampleTime=-1  SaveFormat=Array
  wires:
  In1/1 -> To Workspace/1

== system BD_SER2/generator/ controller <gc>/GC Model/model/enhancedToWorkspace1 ==
  In1 : Inport  Port=1  LatchInput=off
  To Workspace : ToWorkspace  VariableName=gc_trq_in_a  SampleTime=-1  SaveFormat=Array
  wires:
  In1/1 -> To Workspace/1

== system BD_SER2/generator/ controller <gc>/GC Model/model/enhancedToWorkspace2 ==
  In1 : Inport  Port=1  LatchInput=off
  To Workspace : ToWorkspace  VariableName=gc_spd_in_a  SampleTime=-1  SaveFormat=Array
  wires:
  In1/1 -> To Workspace/1

== system BD_SER2/generator/ controller <gc>/GC Model/model/help ==

== system BD_SER2/generator/ controller <gc>/GC Model/model/limit request: controller current limit ==
  computed output power (W) : Inport  Port=1  LatchInput=off
  bus voltage (V) : Inport  Port=2  LatchInput=off
  Block NOTES : Subsystem
      settings: RTWFcnNameOpts=Auto  RTWFileNameOpts=Auto
      mask Display: disp('Block\nNOTES')
  Constant : Constant  Value=gc_max_crrnt
  MinMax : MinMax  Function=min  Inputs=2
  Product1 : Product  Inputs=2  Multiplication=Element-wise(.*)  SaturateOnIntegerOverflow=on
  out_1 : Outport  Port=1  InitialOutput=0
  wires:
  MinMax/1 -> out_1/1
  bus voltage (V)/1 -> Product1/2
  Constant/1 -> Product1/1
  Product1/1 -> MinMax/2
  computed output power (W)/1 -> MinMax/1

== system BD_SER2/motor/controller <mc>/motor model & interface/mc model/Block NOTES ==
  note: Available torque is computed from available power by assuming that the ratio of rotor torque to input
      | (electric) power is the same for the actual/achievable situation as was computed for the request.  This
      | is mathematically equivalent to assuming that the motor/controller efficiency.  Rotor speed for the
      | actual/achievable calculations is as computed in the 'request' branch.
  note: This motor/controller model includes loss data, rotational inertia, and performance limits.

== system BD_SER2/motor/controller <mc>/motor model & interface/mc model/N-m drive torque per W input ==
  req'd input power (W) : Inport  Port=1  LatchInput=off
  req'd rotor drive torque (Nm) : Inport  Port=2  LatchInput=off
  Block NOTES : Subsystem
      settings: RTWFcnNameOpts=Auto  RTWFileNameOpts=Auto
      mask Display: disp('Block\nNOTES')
  Constant : Constant  Value=eps
  Constant1 : Constant  Value=0
  Constant2 : Constant  Value=inf
  Product : Product  Inputs=/*  Multiplication=Element-wise(.*)  SaturateOnIntegerOverflow=on
  Relational Operator : RelationalOperator  Operator=~=
  Sum : Sum  Inputs=++  SaturateOnIntegerOverflow=on
  Switch : Switch  Threshold=eps
  Nm per W : Outport  Port=1  InitialOutput=0
  wires:
  Constant2/1 -> Switch/3
  Constant1/1 -> Relational Operator/2
  req'd input power (W)/1 -> Relational Operator/1, Sum/2
  Sum/1 -> Product/1
  Switch/1 -> Nm per W/1
  Relational Operator/1 -> Switch/2
  Product/1 -> Switch/1
  req'd rotor drive torque (Nm)/1 -> Product/2
  Constant/1 -> Sum/1

== system BD_SER2/motor/controller <mc>/motor model & interface/mc model/documentation10 ==

== system BD_SER2/motor/controller <mc>/motor model & interface/mc model/effect of inertia (Nm) ==
  mc_spd_out_a : Inport  Port=1  LatchInput=off
  Block NOTES : Subsystem
      settings: RTWFcnNameOpts=Auto  RTWFileNameOpts=Auto
      mask Display: disp('Block\nNOTES')
  Constant : Constant  Value=eps
  Constant1 : Constant  Value=max(mc_max_trq)*mc_trq_scale*mc_overtrq_factor
  Constant2 : Constant  Orientation=left  Value=gb_ratio(1)*fd_ratio/wh_radius
  Gain : Gain  Gain=mc_inertia  Multiplication=Element-wise(K.*u)  SaturateOnIntegerOverflow=on
  Memory : Memory  X0=0  InheritSampleTime=off
      settings: RTWStateStorageClass=Auto
  MinMax : MinMax  Function=min  Inputs=2
  Product : Product  Inputs=2  Multiplication=Element-wise(.*)  SaturateOnIntegerOverflow=on
  Sum : Sum  Inputs=++  SaturateOnIntegerOverflow=on
  Switch : Switch  Threshold=eps
  alpha : Derivative
  motor inertia as a function of total vehicle inertia (generous approximation) : Subsystem  Orientation=up
      settings: RTWFcnNameOpts=Auto  RTWFileNameOpts=Auto
  overall gear ratio / wh_radius : Product  Inputs=*/  Multiplication=Element-wise(.*)  SaturateOnIntegerOverflow=on
  out_1 : Outport  Port=1  InitialOutput=0
  wires:
  Switch/1 -> overall gear ratio / wh_radius/2
  Constant2/1 -> Switch/3
  [veh_spd_a_rec_prev] -> Switch/2, Sum/1
  Sum/1 -> Switch/1
  Constant/1 -> Sum/2
  motor inertia as a function of total vehicle inertia (generous approximation)/1(Out1) -> Product/2
  Constant1/1 -> Product/1
  overall gear ratio / wh_radius/1 -> motor inertia as a function of total vehicle inertia (generous approximation)/1(gear ratio)
  Product/1 -> MinMax/2
  Gain/1 -> MinMax/1
  MinMax/1 -> out_1/1
  mc_spd_out_a/1 -> alpha/1, Memory/1
  alpha/1 -> Gain/1
  Memory/1 -> overall gear ratio / wh_radius/1

== system BD_SER2/motor/controller <mc>/motor model & interface/mc model/enforce torque limit ==
  req'd motor torque (Nm) : Inport  Port=1  LatchInput=off
  limited motor speed (rad/s) : Inport  Port=2  LatchInput=off
  Block NOTES : Subsystem
      settings: RTWFcnNameOpts=Auto  RTWFileNameOpts=Auto
      mask Display: disp('Block\nNOTES')
  MinMax : MinMax  Function=min  Inputs=2
  MinMax1 : MinMax  Function=max  Inputs=2
  Relational Operator2 : RelationalOperator  Operator=~=
  Switch : Switch  Threshold=0
  enhancedToWorkspace : Subsystem  mask(enhancedToWorkspace){generalName=generalName, specificName=max_trq_vec, logFlag=logFlag}
      mask prompts: generalName "General Name [char-evaluated]"; specificName "Specific Name [char-literal]"; logFlag "Enable flag (1=on,0=off)"
      mask help: A wrapper for the Simulink "To Workspace" block that allows you to evaluate the name of the variable to log to workspace. This is useful to avoid the double logging errors that occur when you pull in two library models that attempt to log to the same variable.
      mask init:
      | enhancedToWsMaker
      settings: CopyFcn=breakLinkCopyFcn  ParentCloseFcn=breakLinkParCloseFcn  RTWFcnNameOpts=Auto  RTWFileNameOpts=Auto
      mask Help:
      | <h2>Enhanced To Workspace Block</h2>
      | <h3>Parameters</h3>
      | <UL>
      | <li><b>General Name:</b> This is the more general name of the variable. Variables are saved to the workspace as <i>generalName_specificName</i>. Note that this is an evaluated variable. If you would like to type in the value directly, it must be surrounded with single quotes. Otherwise you can input the name of a variable containing a char string.</li>
      | <li><b>Specific Name:</b> This is the specific name of the variable. Note that this is input as a char literal (i.e., you don't need quotes).</li>
      | <li><b>Enable Flag:</b> This flag should have the value of 0 or 1. If 0, the variable will not be logged to the workspace. If 1, the variable will be logged. This is done so that variable logging can be turned off to improve speed.</li>
      | </ul>
      | <h3>Overview</h3>
      | <p>The enhanced to workspace block was put together to allow one to dynamically resolve variable names at run time in simulink. This is most powerful when used in conjunction with a masked subsystem to allow multiple instances of that masked subsytem to be used in the same model. The strategy is to set the generalName in the block mask which will allow the block to change the general name for all variable logging on the fly.
      | <h3>Helper Files</h3>
      | <p>Three m-files are required by the enhancedToWorkspace block. These files are located in the &lt; ADVISOR root &gt;/GUI directory :
      | <ul>
      | <li><i>enhancedToWsMaker.m</i> This file runs the mask initialization for the block</li>
      | <li><i>breakLinkCopyFcn.m</i> This file is used by the block callback when the simulink block is copied. It is necessary to break the link to the enhancedToWorkspace similar to the To Workspace block in order for it to be able to configure itself. (Try copying simulink's To Workspace block--it is impossible to make a link)</li>
      | <li><i>breakLinkParCloseFcn.m</i> This file is similar to the breakLinkCopyFcn and is used when a parent system is closed</li>
      | </ul>
      | <hr>
      | 
      | <p>Created 2003-Jan-21, Michael Patrick O'Keefe, NREL</p>
      mask Display: disp([generalName,'_',specificName])
  max gen torque : Lookup  InputValues=mc_map_spd*mc_spd_scale  OutputValues=mc_max_gen_trq*mc_overtrq_factor*mc_trq_scale
  max torque : Lookup  InputValues=mc_map_spd*mc_spd_scale  OutputValues=mc_max_trq*mc_overtrq_factor*mc_trq_scale
  limited motor torque (Nm) : Outport  Port=1
  tag scope: mc_trq_limited=scoped
  wires:
  max gen torque/1 -> MinMax1/2
  limited motor speed (rad/s)/1 -> max gen torque/1, max torque/1
  Relational Operator2/1 -> [mc_trq_limited]
  MinMax/1 -> Switch/1
  MinMax1/1 -> Switch/3
  Switch/1 -> limited motor torque (Nm)/1, Relational Operator2/2
  req'd motor torque (Nm)/1 -> MinMax/1, MinMax1/1, Switch/2, Relational Operator2/1
  max torque/1 -> enhancedToWorkspace/1(In1), MinMax/2

== system BD_SER2/motor/controller <mc>/motor model & interface/mc model/enhancedToWorkspace ==
  In1 : Inport  Port=1  LatchInput=off
  To Workspace : ToWorkspace  VariableName=mc_pwr_in_a  SampleTime=-1  SaveFormat=Array
  wires:
  In1/1 -> To Workspace/1

== system BD_SER2/motor/controller <mc>/motor model & interface/mc model/enhancedToWorkspace1 ==
  In1 : Inport  Port=1  LatchInput=off
  To Workspace : ToWorkspace  VariableName=mc_ni_trq_out_a  SampleTime=-1  SaveFormat=Array
  wires:
  In1/1 -> To Workspace/1

== system BD_SER2/motor/controller <mc>/motor model & interface/mc model/enhancedToWorkspace2 ==
  In1 : Inport  Port=1  LatchInput=off
  To Workspace : ToWorkspace  VariableName=mc_spd_out_r  SampleTime=-1  SaveFormat=Array
  wires:
  In1/1 -> To Workspace/1

== system BD_SER2/motor/controller <mc>/motor model & interface/mc model/enhancedToWorkspace3 ==
  In1 : Inport  Port=1  LatchInput=off
  To Workspace : ToWorkspace  VariableName=mc_trq_out_r  SampleTime=-1  SaveFormat=Array
  wires:
  In1/1 -> To Workspace/1

== system BD_SER2/motor/controller <mc>/motor model & interface/mc model/enhancedToWorkspace4 ==
  In1 : Inport  Port=1  LatchInput=off
  To Workspace : ToWorkspace  VariableName=mc_pwr_loss  SampleTime=-1  SaveFormat=Array
  wires:
  In1/1 -> To Workspace/1

== system BD_SER2/motor/controller <mc>/motor model & interface/mc model/enhancedToWorkspace5 ==
  In1 : Inport  Port=1  LatchInput=off
  To Workspace : ToWorkspace  VariableName=mc_mc_tmp  SampleTime=-1  SaveFormat=Array
  wires:
  In1/1 -> To Workspace/1

== system BD_SER2/motor/controller <mc>/motor model & interface/mc model/enhancedToWorkspace6 ==
  In1 : Inport  Port=1  LatchInput=off
  To Workspace : ToWorkspace  VariableName=mc_clt_th_pwr  SampleTime=-1  SaveFormat=Array
  wires:
  In1/1 -> To Workspace/1

== system BD_SER2/motor/controller <mc>/motor model & interface/mc model/enhancedToWorkspace7 ==
  In1 : Inport  Port=1  LatchInput=off
  To Workspace : ToWorkspace  VariableName=mc_pwr_in_r  SampleTime=-1  SaveFormat=Array
  wires:
  In1/1 -> To Workspace/1

== system BD_SER2/motor/controller <mc>/motor model & interface/mc model/enhancedToWorkspace8 ==
  In1 : Inport  Port=1  LatchInput=off
  To Workspace : ToWorkspace  VariableName=mc_spd_out_a  SampleTime=-1  SaveFormat=Array
  wires:
  In1/1 -> To Workspace/1

== system BD_SER2/motor/controller <mc>/motor model & interface/mc model/enhancedToWorkspace9 ==
  In1 : Inport  Port=1  LatchInput=off
  To Workspace : ToWorkspace  VariableName=mc_trq_out_a  SampleTime=-1  SaveFormat=Array
  wires:
  In1/1 -> To Workspace/1

== system BD_SER2/motor/controller <mc>/motor model & interface/mc model/mc tmp ==
  Qmc_gen : Inport  Port=1  LatchInput=off
  veh spd : Inport  Port=2  LatchInput=off
  key ON? : Inport  Port=3  LatchInput=off
  Enable : EnablePort  StatesWhenEnabling=reset
  1/mcp : Gain  Gain=1/(mc_mass*mc_cp)  Multiplication=Element-wise(K.*u)  SaturateOnIntegerOverflow=on
  >=0 : Saturate  UpperLimit=Inf  LowerLimit=0  LinearizeAsGain=on
  ">=0 " : Saturate  UpperLimit=Inf  LowerLimit=0  LinearizeAsGain=on
  Block NOTES : Subsystem
      settings: RTWFcnNameOpts=Auto  RTWFileNameOpts=Auto
      mask Display: disp('Block\nNOTES')
  Mux10 : Mux  Inputs=2
      settings: DisplayOption=none
  Mux9 : Mux  Inputs=2
      settings: DisplayOption=none
  Qa : Fcn  Expr=u(1)*(mc_sarea*mc_trq_scale*mc_spd_scale)*u(2)
  Qc1 : Sum  Inputs=-+  SaturateOnIntegerOverflow=on
  Qnet : Sum  Inputs=+++  SaturateOnIntegerOverflow=on
  Qp2a,v7 : Fcn  Expr=amb_tmp-u(1)
  Qr : Fcn  Expr=0.9*(5.67e-8)*(mc_sarea*mc_trq_scale*mc_spd_scale)*((amb_tmp+273)^4 - (u(1)+273)^4)
  Tmc3 : Integrator  ExternalReset=none  InitialConditionSource=internal  InitialCondition=mc_init_tmp  LimitOutput=off  UpperSaturationLimit=inf  LowerSaturationLimit=-inf  ShowSaturationPort=off  ShowStatePort=off  AbsoluteTolerance=auto
  Va/Vv : Gain  Gain=0.5  Multiplication=Element-wise(K.*u)  SaturateOnIntegerOverflow=on
  ha : Fcn  Expr=6 + 6*((abs(u(2))/1000))^0.25 + 60*(abs(u(1))/30)^0.63
  mc coolant : Subsystem  TreatAsAtomicUnit=on
      settings: RTWFcnNameOpts=Auto  RTWFileNameOpts=Auto
  Tmc : Outport  Port=1  InitialOutput=0
  Qmc_clt : Outport  Port=2  OutputWhenDisabled=reset  InitialOutput=0
  wires:
  Qnet/1 -> Qc1/2, mc coolant/2("Qmc ")
  Qc1/1 -> 1/mcp/1
  1/mcp/1 -> Tmc3/1
  Tmc3/1 -> Qp2a,v7/1, Qr/1, Tmc/1, mc coolant/1(Tcl)
  mc coolant/1(Qmc_clt) -> Qc1/1, >=0/1
  >=0/1 -> Qmc_clt/1
  key ON?/1 -> mc coolant/Enable
  veh spd/1 -> Va/Vv/1
  Qa/1 -> Qnet/2
  ">=0 "/1 -> Qnet/1
  Qmc_gen/1 -> ">=0 "/1
  Qr/1 -> Qnet/3
  Qp2a,v7/1 -> Mux10/2, Mux9/2
  ha/1 -> Mux10/1
  Va/Vv/1 -> Mux9/1
  Mux9/1 -> ha/1
  Mux10/1 -> Qa/1

== system BD_SER2/motor/controller <mc>/motor model & interface/mc model/motor controller logic interface ==
  w_mc_out_r : Inport  Port=1  LatchInput=off
  P_mc_in_1lim : Inport  Port=2  LatchInput=off
  motor controller logic : Subsystem
      settings: RTWFcnNameOpts=Auto  RTWFileNameOpts=Auto
  P_mc_in_r : Outport  Port=1  InitialOutput=0
  tag scope: P_mc_in_1lim=scoped, P_mc_in_r=scoped, w_mc_out_r=scoped
  wires:
  w_mc_out_r/1 -> [w_mc_out_r], motor controller logic/3(req'd output spd (rad/s))
  P_mc_in_1lim/1 -> [P_mc_in_1lim], motor controller logic/2(req'd input power (W))
  motor controller logic/1(req'd input power (W)1) -> P_mc_in_r/1, [P_mc_in_r]
  [bus_voltage_prev] -> motor controller logic/1(bus voltage  previous)
  [shifting] -> motor controller logic/4(shifting)
